simulink model "SMC"  (R2018b)
settings: Solver=VariableStepAuto  StartTime=0.0  StopTime=30  RelTol=1e-3
libraries: simulink x2
settings Model: Creator=PV  LastModifiedBy=vudin
settings DataIOCC: ReturnWorkspaceOutputs=on
settings DebuggingCC: UnconnectedInputMsg=none  UnconnectedOutputMsg=none  UnconnectedLineMsg=none  SFMachineParentedDataDiag=error
settings ModelReferenceCC: EnableRefExpFcnMdlSchedulingChecks=off
settings RTWCC: Description=Generic Real-Time Target

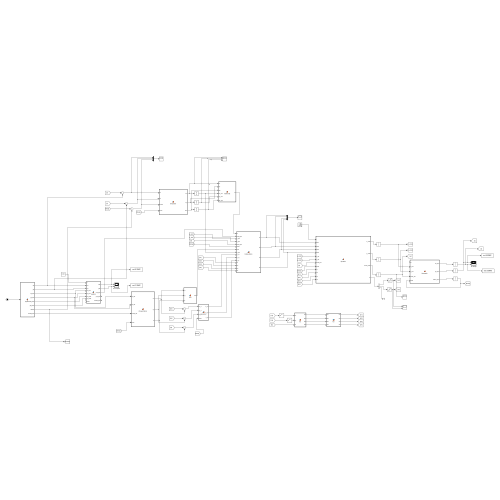
[thumbnail: Simulink's stored preview of the top-level diagram]
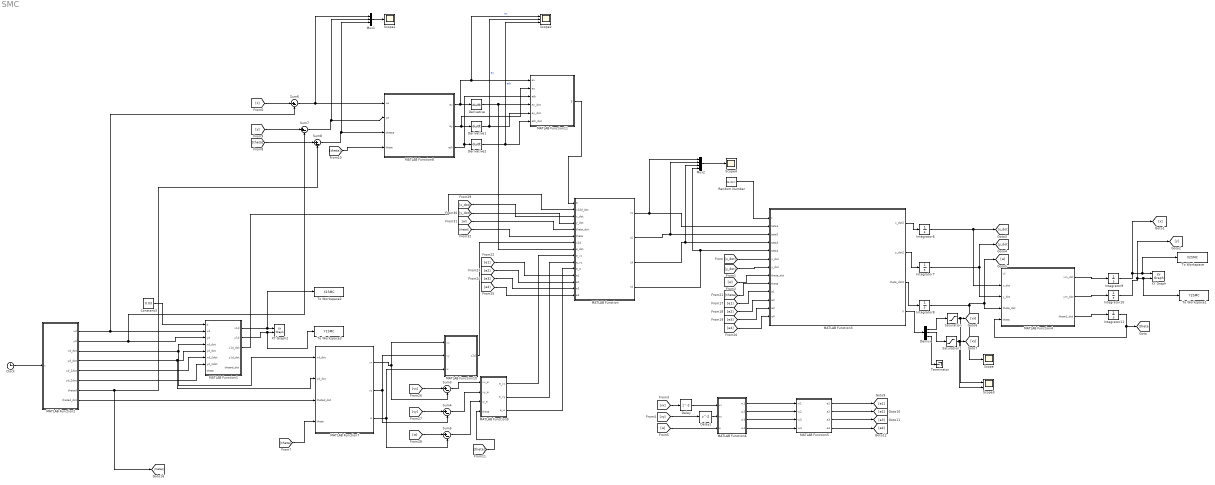
== system SMC ==
  Clock : Clock
  Constant3 : Constant  Value=0.03
  Delay : Delay
  Delay1 : Delay
  Demux : Demux  Outputs=3
  Derivative : Derivative
  Derivative1 : Derivative
  Derivative2 : Derivative
  Integrator{6..10} (5 alike) : Integrator
  Integrator11 : Integrator  InitialCondition=pi/2
  MATLAB Function : MATLAB Function  TreatAsAtomicUnit=on
  MATLAB Function1 : MATLAB Function  TreatAsAtomicUnit=on
  MATLAB Function10 : MATLAB Function  TreatAsAtomicUnit=on
  MATLAB Function11 : MATLAB Function  TreatAsAtomicUnit=on
  MATLAB Function2 : MATLAB Function  TreatAsAtomicUnit=on
  MATLAB Function3 : MATLAB Function  TreatAsAtomicUnit=on
  MATLAB Function4 : MATLAB Function  TreatAsAtomicUnit=on
  MATLAB Function5 : MATLAB Function  TreatAsAtomicUnit=on
  MATLAB Function6 : MATLAB Function  TreatAsAtomicUnit=on
  MATLAB Function7 : MATLAB Function  TreatAsAtomicUnit=on
  MATLAB Function8 : MATLAB Function  TreatAsAtomicUnit=on
  MATLAB Function9 : MATLAB Function  TreatAsAtomicUnit=on
  Mux1 : Mux  Inputs=3
  Mux2 : Mux
  Random Number : RandomNumber  SampleTime=0.1
  Saturation : Saturate  UpperLimit=2  LowerLimit=-2
  Saturation1 : Saturate  UpperLimit=2  LowerLimit=-2
  Scope : Scope
  Scope1 : Scope
  Scope2 : Scope  NumInputPorts=3
  Scope3 : Scope  NumInputPorts=2
  Scope4 : Scope
  Sum{3..8} (6 alike) : Sum  Inputs=|+-
  Terminator : Terminator
  To Workspace : ToWorkspace  VariableName=X2SMC  SampleTime=-1
  To Workspace1 : ToWorkspace  VariableName=Y2SMC  SampleTime=-1
  To Workspace2 : ToWorkspace  VariableName=X1SMC  SampleTime=-1
  To Workspace3 : ToWorkspace  VariableName=Y1SMC  SampleTime=-1
  XY Graph : simulink/Sinks/XY Graph  xmin=-1  xmax=1  ymin=-1  ymax=1  st=-1
  XY Graph2 : simulink/Sinks/XY Graph  xmin=-1  xmax=1  ymin=-1  ymax=1  st=-1
  wires:
  MATLAB Function5/2(e2) -> [e2]
  MATLAB Function5/3(e3) -> [e3]
  [y_dot] -> MATLAB Function3/7(y_dot)
  [w] -> MATLAB Function3/8(theta_dot)
  MATLAB Function5/1(e1) -> [e1]
  [vy] -> Delay1/1
  [theta] -> MATLAB Function7/4(theta)
  Integrator10/1 -> To Workspace1/1, XY Graph/2, [y]
  MATLAB Function2/7(thetad) -> [thetad], Sum8/2
  MATLAB Function4/2(ym_dot) -> Integrator10/1
  Integrator8/1 -> Scope/1, [w], MATLAB Function4/4(theta_dot)
  MATLAB Function2/3(xd_dot) -> MATLAB Function7/1(xd_dot), MATLAB Function1/4(xd_dot)
  MATLAB Function2/1(xd) -> Sum6/2, MATLAB Function1/2(xd)
  MATLAB Function4/1(xm_dot) -> Integrator9/1
  MATLAB Function2/5(xd_2dot) -> MATLAB Function1/6(xd_2dot)
  Clock/1 -> MATLAB Function2/1(t)
  MATLAB Function2/2(yd) -> Sum7/2, MATLAB Function1/3(yd)
  MATLAB Function2/4(yd_dot) -> MATLAB Function7/2(yd_dot), MATLAB Function1/5(yd_dot)
  MATLAB Function6/4(w4) -> MATLAB Function5/4(w4)
  MATLAB Function4/3(theta1_dot) -> Integrator11/1
  MATLAB Function3/2(y_dot2) -> Integrator7/1
  MATLAB Function6/3(w3) -> MATLAB Function5/3(w3)
  MATLAB Function6/1(w1) -> MATLAB Function5/1(w1)
  MATLAB Function3/3(theta_dot2) -> Integrator8/1
  MATLAB Function3/1(x_dot2) -> Integrator6/1
  Sum5/1 -> MATLAB Function9/3(w_e)
  [w] -> Sum5/1
  Sum3/1 -> MATLAB Function9/1(vx_e)
  [vy] -> Sum4/1
  MATLAB Function/4(t4) -> MATLAB Function3/5(teta4), Mux2/4
  [w] -> MATLAB Function/5(theta_dot)
  [thetad] -> MATLAB Function/6(theta)
  MATLAB Function/3(t3) -> Mux2/3, MATLAB Function3/4(teta3)
  Sum4/1 -> MATLAB Function9/2(vy_e)
  [e1] -> MATLAB Function/12(e1)
  Integrator11/1 -> MATLAB Function4/5(theta), [theta]
  [e2] -> MATLAB Function3/11(e2)
  [e1] -> MATLAB Function3/10(e1)
  MATLAB Function1/2(y1d) -> To Workspace3/1, XY Graph2/2
  [e3] -> MATLAB Function3/12(e3)
  MATLAB Function5/4(e4) -> [e4]
  [vx] -> Sum3/1
  MATLAB Function1/1(x1d) -> To Workspace2/1, XY Graph2/1
  [vx] -> Delay/1
  [e4] -> MATLAB Function/15(e4)
  MATLAB Function2/8(thetad_dot) -> MATLAB Function7/3(thetad_dot)
  MATLAB Function/2(t2) -> Mux2/2, MATLAB Function3/3(teta2)
  MATLAB Function6/2(w2) -> MATLAB Function5/2(w2)
  MATLAB Function2/6(yd_2dot) -> MATLAB Function1/7(yd_2dot)
  [e4] -> MATLAB Function3/13(e4)
  [y_dot] -> MATLAB Function/4(y_dot)
  [e2] -> MATLAB Function/13(e2)
  MATLAB Function/1(t1) -> Mux2/1, MATLAB Function3/2(teta1)
  [theta] -> MATLAB Function3/9(theta)
  [w] -> MATLAB Function6/3(w)
  Constant3/1 -> MATLAB Function1/1(b)
  [x_dot] -> MATLAB Function/3(x_dot)
  [x_dot] -> MATLAB Function3/6(x_dot)
  [e3] -> MATLAB Function/14(e3)
  MATLAB Function11/1(S) -> MATLAB Function/1(S)
  Sum8/1 -> Mux1/3, MATLAB Function8/3(thetae)
  [x] -> Sum6/1
  Mux1/1 -> Scope1/1
  Derivative/1 -> MATLAB Function/8(e_dot), MATLAB Function11/4(ex_dot)
  Sum6/1 -> Mux1/1, MATLAB Function8/1(xe)
  MATLAB Function8/3(eth) -> MATLAB Function11/3(eth), Derivative2/1
  MATLAB Function8/2(ey) -> MATLAB Function11/2(ey), Derivative1/1
  Derivative1/1 -> Scope2/2, MATLAB Function11/5(ey_dot)  "ey"
  [theta] -> Sum8/1
  [y] -> Sum7/1
  Derivative2/1 -> Scope2/3, MATLAB Function11/6(eth_dot)  "eth"
  MATLAB Function8/1(ex) -> Scope2/1, MATLAB Function11/1(ex), Derivative/1  "ex"
  Sum7/1 -> Mux1/2, MATLAB Function8/2(ye)
  [theta] -> MATLAB Function8/4(theta)
  MATLAB Function9/1(e_vx) -> MATLAB Function/9(e_vx)
  MATLAB Function9/2(e_vy) -> MATLAB Function/10(e_vy)
  MATLAB Function9/3(e_w) -> MATLAB Function/11(e_w)
  [theta] -> MATLAB Function9/4(theta)
  MATLAB Function7/3(w) -> Sum5/2, MATLAB Function10/3(w)
  MATLAB Function7/1(vx) -> Sum3/2, MATLAB Function10/1(vx)
  MATLAB Function7/2(vy) -> Sum4/2, MATLAB Function10/2(vy)
  MATLAB Function10/1(x2d) -> MATLAB Function/7(x2d)
  MATLAB Function1/3(x1d_dot) -> MATLAB Function/2(x1dd_dot)
  Integrator9/1 -> To Workspace/1, XY Graph/1, [x]
  Random Number/1 -> MATLAB Function3/1(t)
  Mux2/1 -> Scope4/1
  Integrator6/1 -> MATLAB Function4/2(x_dot), [x_dot]
  Integrator7/1 -> MATLAB Function4/3(y_dot), [y_dot]
  MATLAB Function3/4(V) -> Demux/1
  Demux/3 -> Terminator/1
  Demux/2 -> Saturation1/1
  Demux/1 -> Saturation/1
  Delay/1 -> MATLAB Function6/1(vx)
  Delay1/1 -> MATLAB Function6/2(vy)
  Saturation/1 -> Scope3/1, [vx]
  Saturation1/1 -> Scope3/2, [vy]

== matlab function SMC/MATLAB Function1 ==
  data: b input; x1d output; y1d output; x1d_dot output; y1d_dot output; thetad_dot output; xd input; yd input; xd_dot input; yd_dot input; xd_2dot input; yd_2dot input; theta input
function [x1d,y1d,x1d_dot,y1d_dot,thetad_dot] = quydao(b,xd,yd,xd_dot,yd_dot,xd_2dot,yd_2dot,theta)
%% Thiet lap quy dao chuyen dong cho robot
%theta=atan2(yd_dot,xd_dot);
x1d=xd+b*cos(theta);
y1d=yd+b*sin(theta);
wd=(yd_2dot*xd_dot - xd_2dot*yd_dot)/(xd_dot^2+yd_dot^2);
x1d_dot=xd_dot-b*wd*sin(theta);
y1d_dot=yd_dot+b*wd*cos(theta);
thetad_dot=wd;
rot=[cos(theta) 0; sin(theta) 0; 0 1];
p_dot=[xd_dot; yd_dot; wd];
VR=rot\p_dot;

== matlab function SMC/MATLAB Function2 ==
  data: t input; xd output; yd output; xd_dot output; yd_dot output; xd_2dot output; yd_2dot output; thetad output; thetad_dot output
function [xd,yd,xd_dot,yd_dot,xd_2dot,yd_2dot,thetad,thetad_dot] = quydao(t)
%% Khoi tao quy dao chuyen dong
R=5; %ban kinh quy dao
w=0.2; %rad/s =2*pi*f f=w/2/pi -> T=1/f
xd=R*cos(w*t);
yd=R*sin(w*t);
xd_dot=-R*w*sin(w*t);
yd_dot=R*w*cos(w*t);
x0d_dot=-R*w*sin(w);
y0d_dot=R*w*cos(w);
xd_2dot=-R*w^2*cos(w*t);
yd_2dot=-R*w^2*sin(w*t);
theta0=atan2(y0d_dot,x0d_dot)-w;
thetad_dot=w;
thetad=w*t + theta0;

== matlab function SMC/MATLAB Function7 ==
  data: xd_dot input; vx output; yd_dot input; thetad_dot input; theta input; vy output; w output
function [vx,vy,w] = chuyenhetruc(xd_dot,yd_dot,thetad_dot,theta)
H=[cos(theta) -sin(theta) 0; sin(theta) cos(theta) 0; 0 0 1];
P_dot=[xd_dot; yd_dot; thetad_dot];
V=inv(H)*P_dot;
vx=V(1);
vy=V(2);
w=V(3);

== matlab function SMC/MATLAB Function3 ==
  data: t input; teta1 input; x_dot2 output; teta2 input; teta3 input; teta4 input; x_dot input; y_dot input; theta_dot input; y_dot2 output; theta_dot2 output; theta input; e1 input; e2 input; e3 input; e4 input; V output
function [x_dot2,y_dot2,theta_dot2,V] = dynamic(t,teta1,teta2,teta3,teta4,x_dot,y_dot,theta_dot,theta,e1,e2,e3,e4)
m=12;
Ib=0.0032;
r=0.076;
I=6.42*(10^(-4));
l1=0.2;
l2=0.4;


M=[m+(4*Ib)/(r*r) 0 0;0 m+(4*Ib)/(r*r) 0;0 0 I+(4*Ib*(l1+l2)^2)/(r*r)];
C=[m+(4*Ib/(r*r))*y_dot*theta_dot;-m+(4*Ib/(r*r))*x_dot*theta_dot;0];

a=cos(theta);
b=sin(theta);
B=(1/r)*[a+b a-b a+b a-b;-a+b a+b -a+b a+b;-(l1+l2) (l1+l2) (l1+l2) -(l1+l2)];

teta=[teta1;teta2;teta3;teta4];
e=[e1;e2;e3;e4];

q_dot2=pinv(M)*(B*teta-C-B*e);
x_dot2=q_dot2(1);
y_dot2=q_dot2(2);
theta_dot2=q_dot2(3);
%%
rot=[cos(theta) -sin(theta) 0; sin(theta) cos(theta) 0; 0 0 1];
p_dot=[x_dot; y_dot; theta_dot];
V=rot\p_dot;

== matlab function SMC/MATLAB Function4 ==
  data: Ui input; x_dot input; xm_dot output; y_dot input; theta_dot input; theta input; ym_dot output; theta1_dot output
function [xm_dot,ym_dot,theta1_dot] = kinematic(Ui,x_dot,y_dot,theta_dot,theta)

H=[cos(theta) -sin(theta) 0;sin(theta) cos(theta) 0;0 0 1];
q_dot=[x_dot;y_dot;theta_dot];
q2_dot=H*q_dot;
xm_dot=q2_dot(1);
ym_dot=q2_dot(2);
theta1_dot=q2_dot(3);

== matlab function SMC/MATLAB Function5 ==
  data: w1 input; e1 output; w2 input; w3 input; w4 input; e2 output; e3 output; e4 output
function [e1,e2,e3,e4] = fcn(w1,w2,w3,w4)
h=0.2;
r=0.05;
N1=10;
N2=10;
N3=10;
N4=10;
e=[h*r*N1*sign(w1);h*r*N2*sign(w2);h*r*N3*sign(w3);h*r*N4*sign(w4)];
e1=e(1);
e2=e(2);
e3=e(3);
e4=e(4);

== matlab function SMC/MATLAB Function6 ==
  data: vx input; w1 output; vy input; w input; w2 output; w3 output; w4 output
function [w1,w2,w3,w4] = fcn(vx,vy,w)

r=0.05;

l1=2;
l2=2.2;
a=l1+l2;
H=(1/r)*[1 -1 -a;1 1 a;1 -1 a;1 1 -a];
v=[vx;vy;w];
w=H*v;
w1=w(1);
w2=w(2);
w3=w(3);
w4=w(4);

== matlab function SMC/MATLAB Function11 ==
  data: ex input; S output; ey input; eth input; ex_dot input; ey_dot input; eth_dot input
function S = mattruotS(ex,ey,eth,ex_dot,ey_dot,eth_dot)
lamda=[3 0 0;0 3 0;0 0 3];

e1_dot=[ex_dot;ey_dot;eth_dot];
e1=[ex;ey;eth];

S=e1_dot + lamda*e1;

== matlab function SMC/MATLAB Function ==
  data: S input; x1dd_dot input; t1 output; x_dot input; y_dot input; theta_dot input; theta input; x2d input; e_dot input; e_vx input; e_vy input; e_w input; e1 input; e2 input; e3 input; e4 input; t2 output; t3 output; t4 output
function [t1,t2,t3,t4] = bodieukhien(S,x1dd_dot,x_dot,y_dot,theta_dot,theta,x2d,e_dot,e_vx,e_vy,e_w,e1,e2,e3,e4)
m=15;
Ib=0.032;
r=0.075;
I=6.42*(10^(-4));
l1=0.2;
l2=0.4;
k2=10;
T2=0.05;
lamda=[1 0 0;0 1 0;0 0 1];
e2d=[e_vx;e_vy;e_w];

M=[m+(4*Ib)/(r*r) 0 0;0 m+(4*Ib)/(r*r) 0;0 0 I+(4*Ib*(l1+l2)^2)/(r*r)];
C=[m+(4*Ib/(r*r))*y_dot*theta_dot;-m+(4*Ib/(r*r))*x_dot*theta_dot;0];

a=cos(theta);
b=sin(theta);
B=(1/r)*[a+b a-b a+b a-b;-a+b a+b -a+b a+b;-(l1+l2) (l1+l2) (l1+l2) -(l1+l2)];
%T1=[t_dot;t2_dot;t3_dot;t4_dot];
masat=[e1;e2;e3;e4];

T=-B'*pinv(B*B')*(M*(lamda*x2d-x1dd_dot +(k2*sign(S)))-C-B*masat);
t1=T(1);
t2=T(2);
t3=T(3);
t4=T(4);

== matlab function SMC/MATLAB Function9 ==
  data: vx_e input; e_vx output; vy_e input; w_e input; theta input; e_vy output; e_w output
function [e_vx,e_vy,e_w] = loivantoc(vx_e,vy_e,w_e,theta)

A=[cos(theta) sin(theta) 0;
   -sin(theta) cos(theta) 0;
   0 0 1];
B=[vx_e;vy_e;w_e];
C=A*B;

e_vx=C(1);
e_vy=C(2);
e_w=C(3);

== matlab function SMC/MATLAB Function10 ==
  data: vx input; x2d output; vy input; w input
function x2d = x2d(vx,vy,w)

x2d=[vx;vy;w];

== matlab function SMC/MATLAB Function8 ==
  data: xe input; ex output; ye input; thetae input; theta input; ey output; eth output
function [ex,ey,eth] = loiquydao(xe,ye,thetae,theta)

A=[cos(theta) sin(theta) 0;
   -sin(theta) cos(theta) 0;
   0 0 1];
B=[xe;ye;thetae];
C=A*B;

ex=C(1);
ey=C(2);
eth=C(3);
